simulink model "PitchModelReducedOrderObserver"  (R2022a)
settings: Solver=VariableStepAuto  StartTime=0.0  StopTime=100  MaxStep=1e-3  RelTol=1e-6
undefined symbols (not defined in the file): F, G, H
settings Model: Creator=Orkun  LastModifiedBy=Orkun

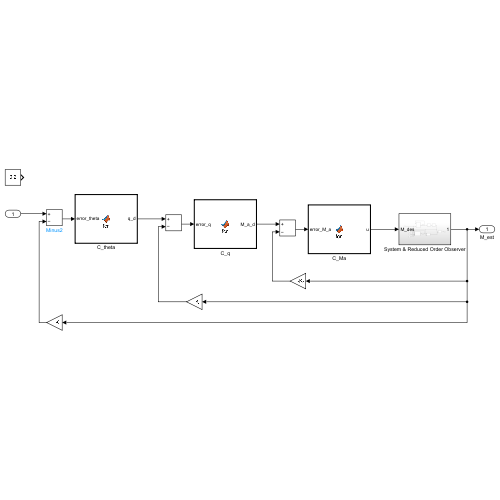
[thumbnail: Simulink's stored preview of the top-level diagram]
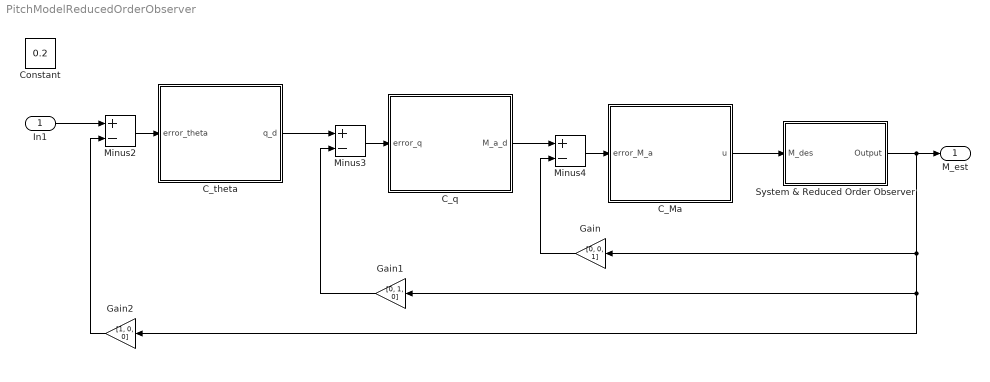
== system PitchModelReducedOrderObserver ==
  In1 : Inport
  C_Ma : MATLAB Function  TreatAsAtomicUnit=on
  C_q : MATLAB Function  TreatAsAtomicUnit=on
  C_theta : MATLAB Function  TreatAsAtomicUnit=on
  Constant : Constant  Value=0.2
  Gain : Gain  Gain=[0, 0, 1]
  Gain1 : Gain  Gain=[0, 1, 0]
  Gain2 : Gain  Gain=[1, 0, 0]
  Minus2 : Sum  Inputs=+-
  Minus3 : Sum  Inputs=+-
  Minus4 : Sum  Inputs=+-
  System & Reduced Order Observer : Subsystem
  M_est : Outport
  wires:
  System & Reduced Order Observer/1(Output) -> Gain2/1, Gain1/1, Gain/1, M_est/1
  Minus2/1 -> C_theta/1(error_theta)
  Minus3/1 -> C_q/1(error_q)
  C_theta/1(q_d) -> Minus3/1
  Minus4/1 -> C_Ma/1(error_M_a)
  C_q/1(M_a_d) -> Minus4/1
  C_Ma/1(u) -> System & Reduced Order Observer/1(M_des)
  Gain/1 -> Minus4/2
  Gain1/1 -> Minus3/2
  Gain2/1 -> Minus2/2
  In1/1 -> Minus2/1

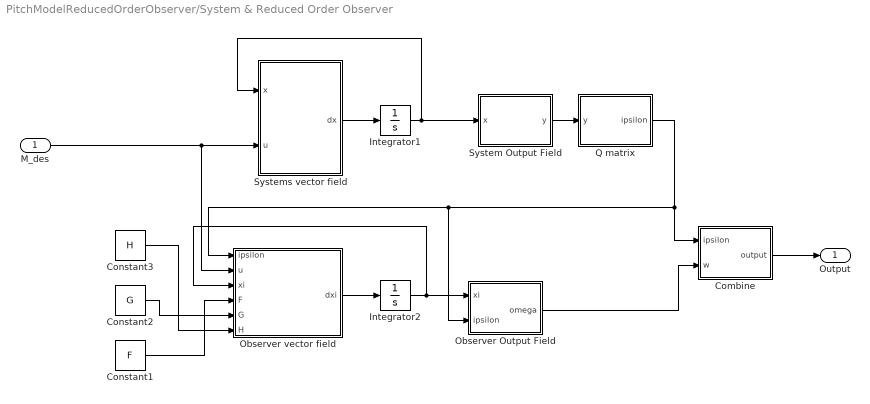
== system PitchModelReducedOrderObserver/System & Reduced Order Observer ==
  M_des : Inport
  Combine : MATLAB Function  TreatAsAtomicUnit=on
  Constant1 : Constant  Value=F
  Constant2 : Constant  Value=G
  Constant3 : Constant  Value=H
  Integrator1 : Integrator  InitialCondition=[0;0;0;0.5]
  Integrator2 : Integrator  InitialCondition=[0;0]
  Observer Output Field : MATLAB Function  TreatAsAtomicUnit=on
  Observer vector field : MATLAB Function  TreatAsAtomicUnit=on
  Q matrix : MATLAB Function  TreatAsAtomicUnit=on
  System Output Field : MATLAB Function  TreatAsAtomicUnit=on
  Systems vector field : MATLAB Function  TreatAsAtomicUnit=on
  Output : Outport
  wires:
  Constant1/1 -> Observer vector field/4(F)
  Systems vector field/1(dx) -> Integrator1/1
  System Output Field/1(y) -> Q matrix/1(y)
  M_des/1 -> Observer vector field/2(u), Systems vector field/2(u)
  Q matrix/1(ipsilon) -> Combine/1(ipsilon), Observer Output Field/2(ipsilon), Observer vector field/1(ipsilon)
  Observer vector field/1(dxi) -> Integrator2/1
  Integrator2/1 -> Observer Output Field/1(xi), Observer vector field/3(xi)
  Constant2/1 -> Observer vector field/5(G)
  Constant3/1 -> Observer vector field/6(H)
  Integrator1/1 -> Systems vector field/1(x), System Output Field/1(x)
  Combine/1(output) -> Output/1
  Observer Output Field/1(omega) -> Combine/2(w)

== matlab function PitchModelReducedOrderObserver/System & Reduced Order Observer/Systems vector field ==
  data: x input; u input; dx output
function dx = fcn(x,u)

A = [0, 1, 0, 0; -11.8336, -0.5779, 358.5000, 1; 0, 0, -33.3333, 0; 0, 0, 0, 0];
B = [0; 0; 33.3333; 0];


dx = (A*x) + (B*u);

== matlab function PitchModelReducedOrderObserver/System & Reduced Order Observer/Combine ==
  data: ipsilon input; output output; w input
function output = fcn(ipsilon, w)

output = [ipsilon;w];

== matlab function PitchModelReducedOrderObserver/System & Reduced Order Observer/System Output Field ==
  data: x input; y output
function y = fcn(x)

C = [1, 0, 0, 0; 0, 1, 0, 0];
y = C*x;

== matlab function PitchModelReducedOrderObserver/System & Reduced Order Observer/Q matrix ==
  data: y input; ipsilon output
function ipsilon = fcn(y)

ipsilon = [1, 0; 0, 1]*y;

== matlab function PitchModelReducedOrderObserver/System & Reduced Order Observer/Observer Output Field ==
  data: xi input; omega output; ipsilon input
function omega = fcn(xi, ipsilon)

L = [0, -0.0475; 0, 2.7];

omega = xi + L*ipsilon;

== matlab function PitchModelReducedOrderObserver/System & Reduced Order Observer/Observer vector field ==
  data: ipsilon input; u input; dxi output; xi input; F input; G input; H input
function dxi = fcn(ipsilon,u, xi, F, G, H)
%F = [-16.3046, 0.0475; -967.95, -2.7];
%F = [-16.3046, 0; -967.9500, 0];
%G = [33.3333; 0];
%H = [-0.5621, 0.8753; 31.9507, 40.2480];
%H = [-0.5621, 0.747; 31.9507, 47.5382];


dxi = F*xi + H*ipsilon + G*u;

== matlab function PitchModelReducedOrderObserver/C_theta ==
  data: error_theta input; q_d output
function q_d = fcn(error_theta)

%TODO: Implement me!
q_d = error_theta;

== matlab function PitchModelReducedOrderObserver/C_q ==
  data: error_q input; M_a_d output
function M_a_d = fcn(error_q)

%TODO: Implement me!
M_a_d = error_q;

== matlab function PitchModelReducedOrderObserver/C_Ma ==
  data: error_M_a input; u output
function u = fcn(error_M_a)

%TODO: Implement me!
u = error_M_a;
